simulink model "gnc_ministack"  (R2025a)
settings: Solver=VariableStepAuto  StartTime=0.0  StopTime=10.0  RelTol=1e-3
settings Model: Creator=Jackt  LastModifiedBy=Jackt

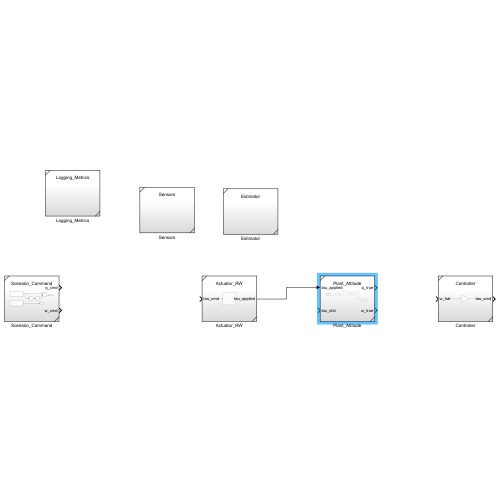
[thumbnail: Simulink's stored preview of the top-level diagram]
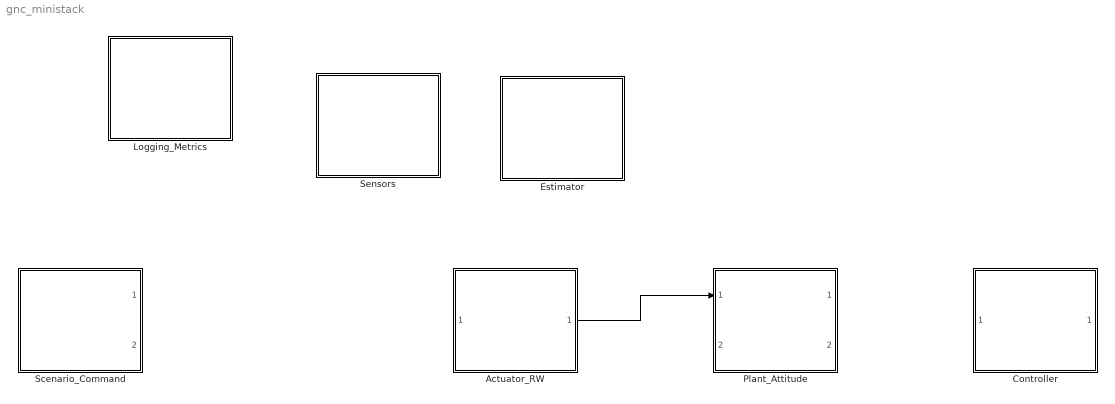
== system gnc_ministack ==
  Actuator_RW : Subsystem  ReferencedSubsystem=Actuator_RW
  Controller : Subsystem  ReferencedSubsystem=Controller
  Estimator : Subsystem  ReferencedSubsystem=Estimator
  Logging_Metrics : Subsystem  ReferencedSubsystem=Logging_Metrics
  Plant_Attitude : Subsystem  ReferencedSubsystem=Plant_Attitude
  Scenario_Command : Subsystem  ReferencedSubsystem=Scenario_Command
  Sensors : Subsystem  ReferencedSubsystem=Sensors
  wires:
  Actuator_RW/1 -> Plant_Attitude/1
